simulink model "HelloWorldContNew"  (Simulink 7.4)
settings: Solver=ode1  StartTime=0.0  StopTime=30  FixedStep=1  MaxStep=1  RelTol=1e-3
undefined symbols (not defined in the file or in its folder): uk, xk
libraries: BLOM_Lib x8, MPCMdlLib x1
settings Model: Creator=vichik  LastModifiedBy=Kyle
settings OptimizationCC: InitFltsAndDblsToZero=on

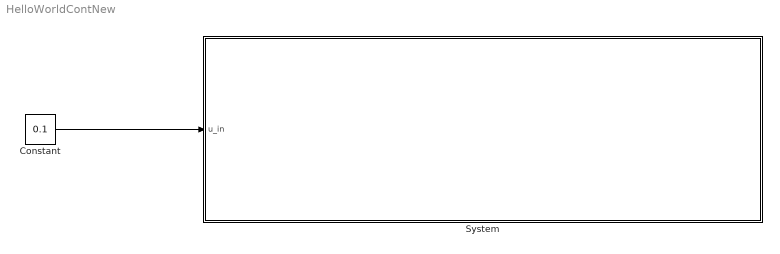
== system HelloWorldContNew ==
  Constant : Constant  Value=0.1
  System : Subsystem
  wires:
  Constant/1 -> System/1(u_in)

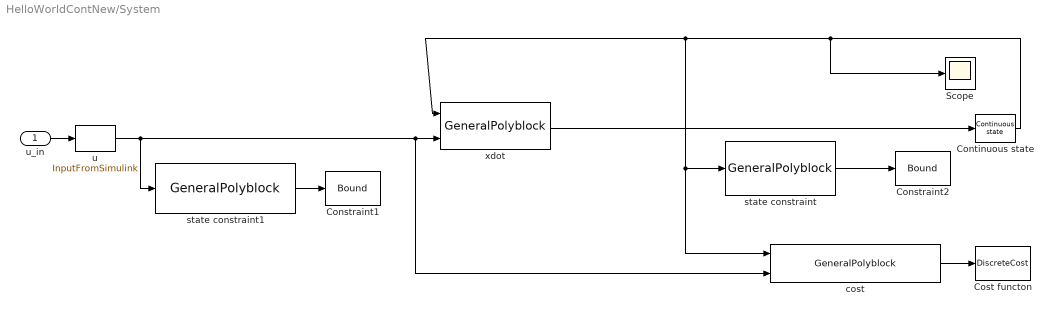
== system HelloWorldContNew/System ==
  u_in : Inport
  Constraint1 : BLOM_Lib/Bound  SystemSampleTime=-1  ub=0  lb=-inf  initial_step=on  final_step=on  intermediate_step=on
  Constraint2 : BLOM_Lib/Bound  SystemSampleTime=-1  ub=0  lb=-inf  initial_step=on  final_step=on  intermediate_step=on
  Continuous state : MPCMdlLib/Continuous state  Tag=OptState  SystemSampleTime=-1  init_val=0.6  save_name=BL_System_Continuous_state
  Cost functon : BLOM_Lib/DiscreteCost  SystemSampleTime=-1  initial_step=on  final_step=on  intermediate_step=on
  Scope : Scope
  "cost " : BLOM_Lib/GeneralPolyblock  SystemSampleTime=-1  P_f=[2 0; 0 2]  K_f=[0.5 2]  P_g=[0 0 ]  K_g=1  inputs=xk,uk  inputScalar=on  outputScalar=on
  state constraint : BLOM_Lib/GeneralPolyblock  SystemSampleTime=-1  P_f="[1  ;  0 ]"  K_f=[1 -1 ; -1 0.5 ]  P_g="[0  ]"  K_g=1  inputs=x  inputScalar=on  outputScalar=off
  state constraint1 : BLOM_Lib/GeneralPolyblock  SystemSampleTime=-1  P_f="[1  ;  0 ]"  K_f=[1 -2 ; -1 -2 ]  P_g="[0  ]"  K_g=1  inputs=u  inputScalar=on  outputScalar=off
  u : BLOM_Lib/InputFromSimulink  SystemSampleTime=-1  interpType=Zero-Order Hold
  xdot : BLOM_Lib/GeneralPolyblock  SystemSampleTime=-1  P_f=[1 0; 0 1]  K_f=[-0.1 1]  P_g=[0 0 ]  K_g=1  inputs=xk,uk  inputScalar=on  outputScalar=on
  wires:
  xdot/1 -> Continuous state/1
  Continuous state/1 -> xdot/1, state constraint/1, "cost "/1, Scope/1
  u/1 -> xdot/2, "cost "/2, state constraint1/1
  "cost "/1 -> Cost functon/1
  state constraint/1 -> Constraint2/1
  u_in/1 -> u/1
  state constraint1/1 -> Constraint1/1
